simulink model "DCDC_12_5"  (R2014a)
settings: Solver=ode45  StartTime=0.0  StopTime=100  FixedStep=0.001  MaxStep=0.005  RelTol=1e-3
undefined symbols (not defined in the file): Ion, Lithium
libraries: powerlib x9, electricdrivelib x2
settings Model: Creator=Administrator  LastModifiedBy=Administrator
settings SolverCC: AlgebraicLoopSolver=LineSearch
settings DataIOCC: SignalLoggingSaveFormat=ModelDataLogs
settings OptimizationCC: ExpressionDepthLimit=2147483647
settings DebuggingCC: UnderspecifiedInitializationDetection=Classic  FcnCallInpInsideContextMsg=UseLocalSettings  StateNameClashWarn=warning
settings GRTTargetCC: CombineOutputUpdateFcns=off  GRTInterface=on

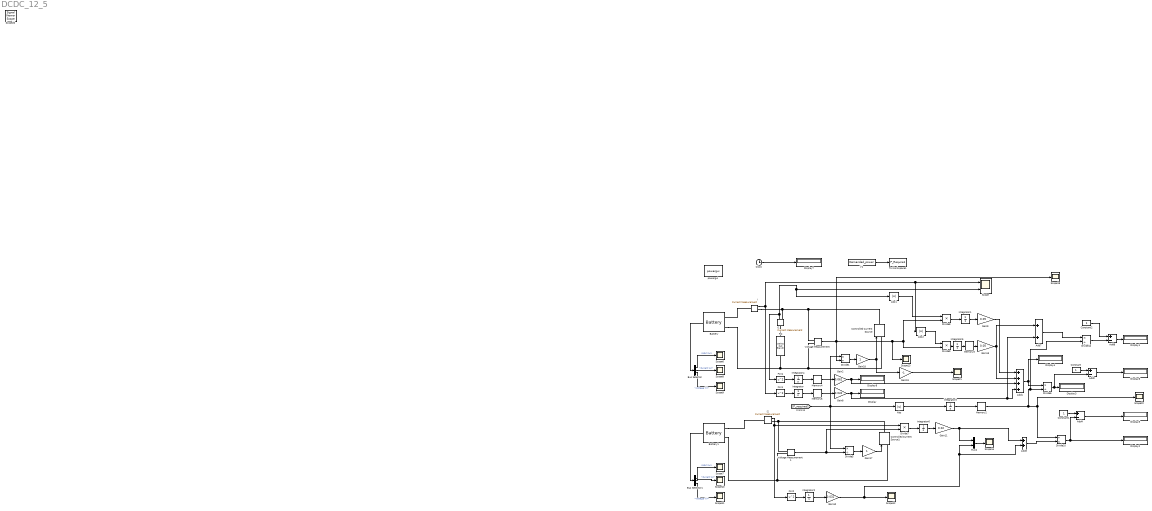
== system DCDC_12_5 ==
  Abs : Abs
  Abs1 : Abs
  Abs2 : Abs
  Add1 : Sum  Inputs=++++
  Add2 : Sum  Inputs=+-
  Add3 : Sum
  Add4 : Sum  Inputs=+-
  Add7 : Sum
  Add8 : Sum  Inputs=+-
  Battery : electricdrivelib/Extra Sources/Battery  BatType=Lithium-Ion  ShowDetailedParameters=on  NomV=576  NomQ=180  SOC=90  PresetModel=off  MaxQ=180  FullV=670.4566  Dis_rate=78.2609  R=0.032  Normal_OP=162.7826  expZone="[622.3023      8.843478]"  Dis_Char=off  current=[1.5 3]  Units=Ampere-hour  Batt_Tr=30
  Battery1 : electricdrivelib/Extra Sources/Battery  BatType=Lithium-Ion  ShowDetailedParameters=on  NomV=576  NomQ=180  SOC=90  PresetModel=off  MaxQ=180  FullV=670.4566  Dis_rate=78.2609  R=0.032  Normal_OP=162.7826  expZone="[622.3023      8.843478]"  Dis_Char=off  current=[1.5 3]  Units=Ampere-hour  Batt_Tr=30
  Bus Selector : BusSelector  OutputSignals=SOC (%),Current (A),Voltage (V)
  Bus Selector1 : BusSelector  OutputSignals=SOC (%),Current (A),Voltage (V)
  Clock : Clock
  Constant : Constant
  Constant1 : Constant
  Constant2 : Constant
  Controlled Current Source : powerlib/Electrical Sources/Controlled Current Source  Initialize=on  Source_Type=AC  Amplitude=0  Phase=0  Frequency=0  Measurements=None
  Controlled Current Source1 : powerlib/Electrical Sources/Controlled Current Source  Initialize=on  Source_Type=AC  Amplitude=0  Phase=0  Frequency=0  Measurements=None
  Display{,1..8} (9 alike) : Display
  Divide{1,5..6,12} (4 alike) : Product  Inputs=*/
  Divide10 : Product  Inputs=/*
  Divide7 : Product  Inputs=**
  Divide8 : Product  Inputs=**
  Divide9 : Product  Inputs=**
  Fcn1 : Fcn  Expr=u^2
  Fcn2 : Fcn  Expr=u^2
  Fcn4 : Fcn  Expr=u^2
  Gain10 : Gain  Gain=0.032
  Gain11 : Gain  Gain=0.02
  Gain13 : Gain  Gain=0.05
  Gain17 : Gain
  Gain18 : Gain
  Gain19 : Gain  Gain=-1
  Gain2 : Gain  Gain=0.062
  Gain8 : Gain  Gain=0.032
  Gain9 : Gain  Gain=0.05
  I : powerlib/Measurements/Current Measurement  PhasorSimulation=off  OutputType=Complex  PSBequivalent=0
  I1 : powerlib/Measurements/Current Measurement  PhasorSimulation=off  OutputType=Complex  PSBequivalent=0
  I2 : powerlib/Measurements/Current Measurement  PhasorSimulation=off  OutputType=Complex  PSBequivalent=0
  Integrator{,1..2,4..6} (6 alike) : Integrator
  Integrator3 : Integrator  InitialCondition=1
  Memory{2..5} (4 alike) : Memory
  Mux2 : Mux  Inputs=2
  RC : powerlib/Elements/Series RLC Branch  LConnTagsString=__new0  RConnTagsString=__new0  BranchType=RC  Resistance=0.062  Inductance=1e-3  SetiL0=off  InitialCurrent=0  Capacitance=14.0845  Setx0=on  InitialVoltage=576  Measurements=None
  Scope : Scope  NumInputPorts=2
      settings: YMin=-5~-5  YMax=5~5  SaveName=ScopeData5
  Scope{6..14,19,21..22} (12 alike) : Scope
      Scope10 settings: SaveName=ScopeData9
      Scope11 settings: SaveName=ScopeData13
      Scope12 settings: SaveName=ScopeData15
      Scope13 settings: SaveName=ScopeData16
      Scope14 settings: YMin=34000  YMax=55000  SaveName=ScopeData17
      Scope19 settings: SaveName=ScopeData22
      Scope21 settings: SaveName=ScopeData23
      Scope22 settings: SaveName=ScopeData24
      Scope6 settings: SaveName=ScopeData7
      Scope7 settings: SaveName=ScopeData14
      Scope8 settings: SaveName=ScopeData11
      Scope9 settings: SaveName=ScopeData12
  To Workspace1 : ToWorkspace  VariableName=P_Require1  SampleTime=-1
  V1 : FromWorkspace  VariableName=Demanded_power  SampleTime=1
  Voltage Measurement : powerlib/Measurements/Voltage Measurement  PhasorSimulation=off  OutputType=Complex  PSBequivalent=0
  Voltage Measurement1 : powerlib/Measurements/Voltage Measurement  PhasorSimulation=off  OutputType=Complex  PSBequivalent=0
  powergui : powerlib/powergui  Priority=1  SimulationMode=Discrete  SolverType=Tustin  SampleTime=0.01  frequency=60  SPID=off  DisableSnubberDevices=off  DisableRonSwitches=off  DisableVfSwitches=off  SwTol=0  Interpol=off  DisplayEquations=off  Ts=0  methode=off  frequencyindice=0  Pbase=100e6  ErrMax=1e-4  Iterations=50  UnitsV=kV  UnitsW=MW  FunctionMessages=off  echomessages=off  HookPort=off  EnableUseOfTLC=off  x0status=blocks  RestoreLinks=warning  ResistiveCurrentMeasurement=off  Frange=[0:2:500]  Ylog=off  Xlog=on  ShowGrid=off  save=off  variable=ZData  structure=0  ZoomFFT=off  StartTime=0.0  cycles=1  DisplayStyle=1  fundamental=60  FreqAxis=off  MaxFrequency=1000  frequencyindicesteady=1  RmsSteady=1  display=off
  Scope20 : SignalViewerScope  IOType=viewer  RefreshTime=0.035000
  wires:
  I/1 -> Abs2/1, Scope/1, Fcn1/1
  Voltage Measurement/1 -> Scope19/1, Scope13/1, Divide9/2, Divide8/2, Divide1/2
  Divide1/1 -> Gain18/1
  Fcn1/1 -> Integrator/1
  Integrator/1 -> Memory5/1
  Gain8/1 -> Add7/2, Add1/4, Display/1
  Integrator1/1 -> Gain9/1
  Gain9/1 -> Add1/1
  Divide6/1 -> Display3/1, Add2/2
  Add1/1 -> Display4/1, Divide6/1
  Integrator3/1 -> Memory2/1
  Constant/1 -> Add2/1
  Add2/1 -> Display6/1
  Abs/1 -> Integrator3/1
  Fcn4/1 -> Integrator4/1
  Integrator4/1 -> Memory4/1
  Gain2/1 -> Add1/3, Display8/1
  Battery/1 -> Bus Selector/1
  Bus Selector/1 -> Scope6/1  "<SOC (%)>"
  Bus Selector/2 -> Scope8/1  "<Current (A)>"
  Bus Selector/3 -> Scope9/1  "<Voltage (V)>"
  Abs1/1 -> Divide8/1
  Divide8/1 -> Integrator1/1
  Divide9/1 -> Integrator5/1
  Gain13/1 -> Add1/2, Add7/1
  Abs2/1 -> Divide9/1
  I1/1 -> Fcn4/1, Abs1/1, Scope/2
  Add7/1 -> Divide12/1
  Divide12/1 -> Add8/2
  Constant2/1 -> Add8/1
  Add8/1 -> Display1/1
  Memory2/1 -> Scope22/1, Divide10/1, Divide12/2, Divide6/2
  Integrator5/1 -> Memory3/1
  Memory3/1 -> Gain13/1
  Memory4/1 -> Gain2/1
  Memory5/1 -> Gain8/1
  [P_required] -> Abs/1, Divide5/1, Divide1/1
  Battery1/1 -> Bus Selector1/1
  Bus Selector1/1 -> Scope7/1  "<SOC (%)>"
  Bus Selector1/2 -> Scope10/1  "<Current (A)>"
  Bus Selector1/3 -> Scope11/1  "<Voltage (V)>"
  Voltage Measurement1/1 -> Divide7/2, Divide5/2
  Divide5/1 -> Gain17/1
  Fcn2/1 -> Integrator2/1
  I2/1 -> Divide7/1, Fcn2/1
  Integrator2/1 -> Gain10/1
  Gain10/1 -> Add3/2, Mux2/2, Scope12/1
  Integrator6/1 -> Gain11/1
  Divide7/1 -> Integrator6/1
  Gain11/1 -> Add3/1, Mux2/1
  Mux2/1 -> Scope14/1
  Gain17/1 -> Controlled Current Source1/1
  Gain18/1 -> Gain19/1, Controlled Current Source/1
  Add3/1 -> Divide10/2
  Divide10/1 -> Add4/2, Display2/1
  Constant1/1 -> Add4/1
  Add4/1 -> Display5/1
  Gain19/1 -> Scope21/1
  Clock/1 -> Display7/1
  V1/1 -> To Workspace1/1
  connections:
  I/RConn1 -- I1/RConn1 -- Controlled Current Source/RConn1 -- Voltage Measurement/LConn1
  RC/RConn1 -- Controlled Current Source/LConn1 -- Voltage Measurement/LConn2 -- Battery/LConn2
  I/LConn1 -- Battery/LConn1
  RC/LConn1 -- I1/LConn1
  Battery1/LConn1 -- I2/LConn1
  Controlled Current Source1/RConn1 -- Voltage Measurement1/LConn1 -- I2/RConn1
  Battery1/LConn2 -- Voltage Measurement1/LConn2 -- Controlled Current Source1/LConn1
